simulink model "mdl_with_State_Feedback_integrale"  (R2025b)
settings: Solver=FixedStepAuto  StartTime=0.0  StopTime=Tsim  FixedStep=Ts  RelTol=1e-3
values from neighbouring files (symbols this model uses):
  g = 9.81    [exo.m]    (also in parameters.m = 9.82; test_anime.m = params.g)
  IC = [0,deg2rad(1),0,0]    [Copy_of_main_final.m]
  k1 = 0.01    [parameters.m]
  k2 = 0.01    [parameters.m]
  l = params.l    [animate_pendulum_cart.m]    (also in animate_pendulum_cart_wheel_.m = params.L; exo.m = 1; parameters.m = 1)
  M = 1.5    [parameters.m]
  m = 0.5    [parameters.m]
  plant_ss = plant_ss_q1    [Copy_of_main_final.m]    (also in syst_repr_generator.m = ss(A,B,C,D))
  plant_ss_diag = diagonalize(plant_ss)    [Copy_of_main_final.m]    (also in diagonalize.m = ss(A_d, B_d, C_d, 0))
  q2_f = deg2rad(10)    [Copy_of_main_final.m]
libraries: SignalEditorBlockLib x1
settings Model: Creator=dsagn  LastModifiedBy=dsagn
settings SolverCC: AlgebraicLoopSolver=TrustRegion
settings DataIOCC: ReturnWorkspaceOutputs=off
settings DebuggingCC: UnconnectedInputMsg=warning  UnconnectedOutputMsg=warning  UnconnectedLineMsg=warning  ArithmeticOperatorsInVariantConditions=warning
settings ModelReferenceCC: EnableRefExpFcnMdlSchedulingChecks=on
settings SFSimCC: CustomCodeUndefinedFunction=UseInterfaceOnly
settings RTWCC: GPUComputeCapability=3.5

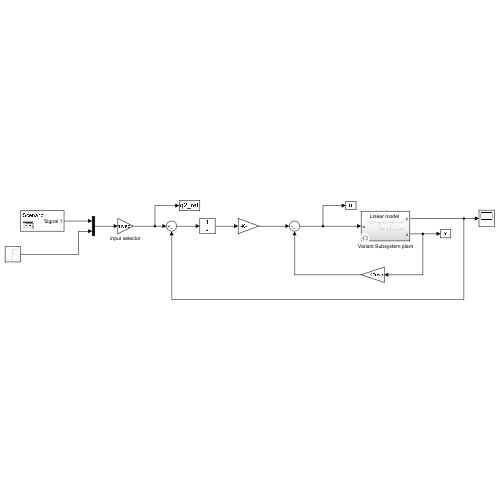
[thumbnail: Simulink's stored preview of the top-level diagram]
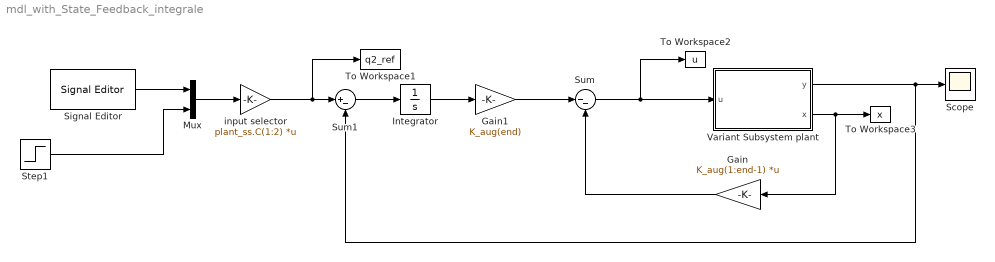
== system mdl_with_State_Feedback_integrale ==
  Gain : Gain  Gain=K_aug(1:end-1)  Multiplication=Matrix(K*u) (u vector)
  Gain1 : Gain  Gain=K_aug(end)
  Integrator : Integrator
  Mux : Mux  Inputs=2
  Scope : Scope
      settings: ActiveDisplayYMinimum=-1  ActiveDisplayYMaximum=1
  Signal Editor : SignalEditorBlockLib/Signal Editor  FileName=q1_scenario1.mat  ActiveScenario=Scenario  ActiveSignal=Signal 1  IsBus=off  OutputBusObjectStr=Bus: BusObject  SampleTime=0  ZeroCross=off  OutputAfterFinalValue=Setting to zero  Unit=inherit  PreserveSignalName=on  ApplySigPropsToAllScenarios=on  ApplySigPropsToAllSignals=off  SignalPropertySource=Dialog parameters
  Step1 : Step  After=q2_f  SampleTime=0
  Sum : Sum  Inputs=|--
  Sum1 : Sum  Inputs=|+-
  To Workspace1 : ToWorkspace  VariableName=q2_ref  SaveFormat=Timeseries  SampleTime=-1
  To Workspace2 : ToWorkspace  VariableName=u  SaveFormat=Timeseries  SampleTime=-1
  To Workspace3 : ToWorkspace  VariableName=x  SaveFormat=Timeseries  SampleTime=-1
  Variant Subsystem plant : Subsystem  Variant=on
  input selector : Gain  Gain=plant_ss.C(1:2)  Multiplication=Matrix(K*u) (u vector)
  wires:
  Sum/1 -> Variant Subsystem plant/1(u), To Workspace2/1
  Variant Subsystem plant/2(x) -> To Workspace3/1, Gain/1
  Gain/1 -> Sum/2
  Sum1/1 -> Integrator/1
  input selector/1 -> Sum1/1, To Workspace1/1
  Variant Subsystem plant/1(y) -> Scope/1, Sum1/2
  Integrator/1 -> Gain1/1
  Gain1/1 -> Sum/1
  Mux/1 -> input selector/1
  Step1/1 -> Mux/2
  Signal Editor/1 -> Mux/1

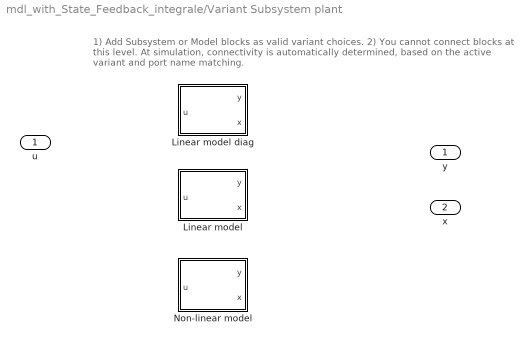
== system mdl_with_State_Feedback_integrale/Variant Subsystem plant ==
  note: 1) Add Subsystem or Model blocks as valid variant choices.
      | 2) You cannot connect blocks at this level. At simulation, connectivity is automatically
      | determined, based on the active variant and port name matching.
  u : Inport
  "Linear model " : Subsystem  VariantControl=model==1
  Linear model diag : Subsystem  VariantControl=model==2
  Non-linear model : Subsystem  VariantControl=model==3
  y : Outport
  x : Outport  Port=2

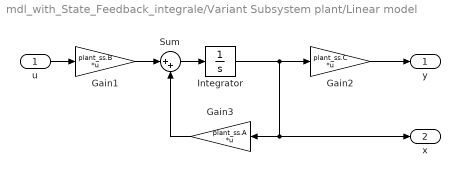
== system mdl_with_State_Feedback_integrale/Variant Subsystem plant/Linear model  ==
  u : Inport
  Gain1 : Gain  Gain=plant_ss.B  Multiplication=Matrix(K*u) (u vector)
  Gain2 : Gain  Gain=plant_ss.C  Multiplication=Matrix(K*u) (u vector)
  Gain3 : Gain  Gain=plant_ss.A  Multiplication=Matrix(K*u) (u vector)
  Integrator : Integrator  InitialCondition=IC
  Sum : Sum  Inputs=|++
  y : Outport
  x : Outport  Port=2
  wires:
  u/1 -> Gain1/1
  Gain1/1 -> Sum/1
  Sum/1 -> Integrator/1
  Gain3/1 -> Sum/2
  Integrator/1 -> Gain2/1, Gain3/1, x/1
  Gain2/1 -> y/1

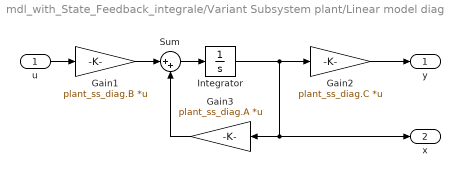
== system mdl_with_State_Feedback_integrale/Variant Subsystem plant/Linear model diag ==
  u : Inport
  Gain1 : Gain  Gain=plant_ss_diag.B  Multiplication=Matrix(K*u) (u vector)
  Gain2 : Gain  Gain=plant_ss_diag.C  Multiplication=Matrix(K*u) (u vector)
  Gain3 : Gain  Gain=plant_ss_diag.A  Multiplication=Matrix(K*u) (u vector)
  Integrator : Integrator  InitialCondition=IC
  Sum : Sum  Inputs=|++
  y : Outport
  x : Outport  Port=2
  wires:
  Gain2/1 -> y/1
  Integrator/1 -> x/1, Gain3/1, Gain2/1
  Gain3/1 -> Sum/2
  Sum/1 -> Integrator/1
  Gain1/1 -> Sum/1
  u/1 -> Gain1/1

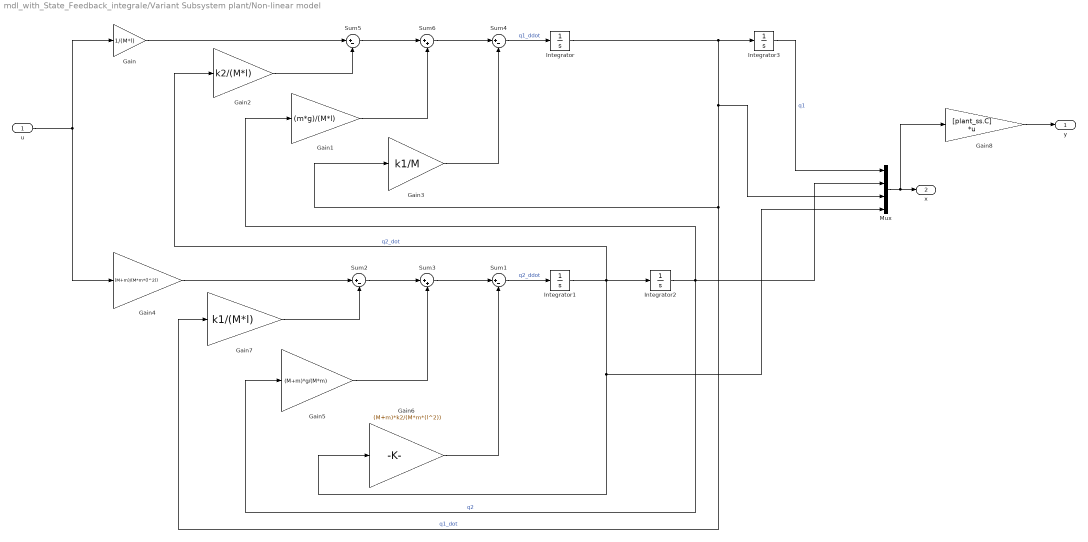
== system mdl_with_State_Feedback_integrale/Variant Subsystem plant/Non-linear model ==
  "u " : Inport
  Gain : Gain  Gain=1/(M*l)
  Gain1 : Gain  Gain=(m*g)/(M*l)
  Gain2 : Gain  Gain=k2/(M*l)
  Gain3 : Gain  Gain=k1/M
  Gain4 : Gain  Gain=(M+m)/(M*m*(l^2))
  Gain5 : Gain  Gain=(M+m)*g/(M*m)
  Gain6 : Gain  Gain=(M+m)*k2/(M*m*(l^2))
  Gain7 : Gain  Gain=k1/(M*l)
  Gain8 : Gain  Gain=[plant_ss.C]  Multiplication=Matrix(K*u) (u vector)
  Integrator : Integrator
  Integrator1 : Integrator
  Integrator2 : Integrator  InitialCondition=IC(2)
  Integrator3 : Integrator
  Mux : Mux
  Sum{1..2,4..5} (4 alike) : Sum  Inputs=|+-
  Sum3 : Sum  Inputs=|++
  Sum6 : Sum  Inputs=|++
  y : Outport  VectorParamsAs1DForOutWhenUnconnected=off
  x : Outport  Port=2
  wires:
  Sum4/1 -> Integrator/1  "q1_ddot"
  "u "/1 -> Gain4/1, Gain/1
  Gain1/1 -> Sum6/2
  Gain2/1 -> Sum5/2
  Gain3/1 -> Sum4/2
  Integrator/1 -> Integrator3/1, Mux/3, Gain7/1, Gain3/1  "q1_dot"
  Gain4/1 -> Sum2/1
  Gain5/1 -> Sum3/2
  Gain6/1 -> Sum1/2
  Gain7/1 -> Sum2/2
  Sum1/1 -> Integrator1/1  "q2_ddot"
  Integrator1/1 -> Mux/4, Gain6/1, Gain2/1, Integrator2/1  "q2_dot"
  Integrator2/1 -> Mux/2, Gain5/1, Gain1/1  "q2"
  Sum2/1 -> Sum3/1
  Sum3/1 -> Sum1/1
  Sum6/1 -> Sum4/1
  Gain/1 -> Sum5/1
  Sum5/1 -> Sum6/1
  Integrator3/1 -> Mux/1  "q1"
  Mux/1 -> Gain8/1, x/1
  Gain8/1 -> y/1
